simulink model "carTransStart"  (R2020a)
settings: Solver=ode23t  StartTime=0.0  StopTime=30  RelTol=1e-3  AbsTol=1e-3  EnableMultiTasking=on
libraries: nesl_utility x20, fl_lib x20, sdl_lib x17, simulink x1
settings Model: FPTRunName=Active  ExtModeAutoUpdateStatusClock=off  Creator=MathWorks  LastModifiedBy=SIDD N
settings SolverCC: AutoScaleAbsTol=off  ZcThreshold=0  ZeroCrossAlgorithm=Adaptive
settings DataIOCC: LimitDataPoints=on  SaveFormat=Array  SignalLoggingSaveFormat=ModelDataLogs  SaveOutput=off  SignalLogging=off  DSMLogging=off  SaveTime=off  ReturnWorkspaceOutputs=off
settings OptimizationCC: ExpressionDepthLimit=2147483647  InitFltsAndDblsToZero=on  LifeSpan=inf  BufferReusableBoundary=off
settings DebuggingCC: SaveWithParameterizedLinksMsg=none  UnderspecifiedInitializationDetection=Classic  MergeDetectMultiDrivingBlocksExec=none  SignalResolutionControl=TryResolveAllWithWarning  MultiTaskDSMMsg=warning  MultiTaskCondExecSysMsg=none  SigSpecEnsureSampleTimeMsg=none  FcnCallInpInsideContextMsg=warning  BusObjectLabelMismatch=none  StateNameClashWarn=warning  SFUnexpectedBacktrackingDiag=warning  SFNoUnconditionalDefaultTransitionDiag=warning  SFExecutionAtInitializationDiag=none  ArithmeticOperatorsInVariantConditions=warning
settings HardwareCC: ProdBitPerPointer=32  ProdBitPerSizeT=32  ProdBitPerPtrDiffT=32  ProdLargestAtomicFloat=None  ProdIntDivRoundTo=Undefined  ProdEndianess=Unspecified  ProdWordSize=32  ProdHWDeviceType=32-bit Generic  TargetBitPerPointer=64  TargetBitPerSizeT=64  TargetBitPerPtrDiffT=64  TargetLongLongMode=on  TargetIntDivRoundTo=Zero  TargetEndianess=LittleEndian  TargetWordSize=64  TargetHWDeviceType=MATLAB Host  ProdEqTarget=off
settings ModelReferenceCC: PropagateSignalLabelsOutOfModel=off
settings SFSimCC: SimUseLocalCustomCode=off  CustomCodeUndefinedFunction=UseInterfaceOnly
settings RTWCC: Description=Generic Real-Time Target  RTWUseLocalCustomCode=off
settings CodeAppCC: StateflowObjectComments=on
settings GRTTargetCC: TargetLangStandard=C89/C90 (ANSI)  CombineOutputUpdateFcns=off  GRTInterface=on
settings ConfigComp: CovMetricSettings=dw  CovHtmlReporting=on  CovSaveCumulativeToWorkspaceVar=on  CovSaveSingleToWorkspaceVar=on  CovExternalEMLEnable=off  CovSFcnEnable=off
settings SimscapeCC: SimscapeNormalizeSystem=off

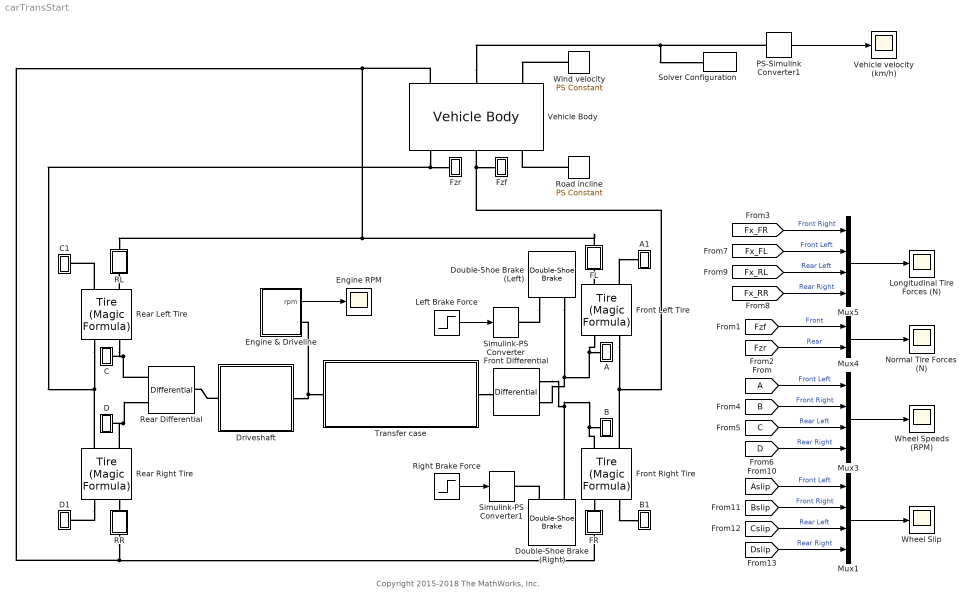
== system carTransStart ==
  note: Copyright 2015-2018 The MathWorks, Inc.
  A : Subsystem
  A1 : Subsystem
  B : Subsystem
  B1 : Subsystem
  C : Subsystem
  C1 : Subsystem
  D : Subsystem
  D1 : Subsystem
  Double-Shoe Brake (Left) : sdl_lib/Brakes & Detents/Rotational/Double-Shoe Brake  r_drum=200 mm  r_act=150 mm  r_pin=125 mm  theta_pin=15 deg  theta_0=5 deg  theta_shoe=120 deg  mu_visc=.01 N*m/(rad/s)  thermal_port=simscape.enum.thermaleffects.omit  mu=0.3  temperature_TLU=[280, 300, 320] K  mu_TLU=[.1, .05, .03]  thermal_mass=50 kJ/K  w_thr=0.01 rad/s  temperature_specify=off  temperature_priority=High  temperature=300 K  temperature_nominal_specify=off  temperature_nominal_unit=K  temperature_nominal_value=1
      settings: SourceProductBaseCode=LD  InternalSimscapePortConfiguration="{\"Bottom\":[],\"Left\":[{\"id\":\"F\",\"label\":\"F\",\"type\":\"input\"},{\"id\":\"S\",\"label\":\"S\",\"type\":\"foundation.mechanical.rotational.rotational\"}],\"Right\":[],\"Top\":[]}"
  Double-Shoe Brake (Right) : sdl_lib/Brakes & Detents/Rotational/Double-Shoe Brake  r_drum=200 mm  r_act=150 mm  r_pin=125 mm  theta_pin=15 deg  theta_0=5 deg  theta_shoe=120 deg  mu_visc=.01 N*m/(rad/s)  thermal_port=simscape.enum.thermaleffects.omit  mu=0.3  temperature_TLU=[280, 300, 320] K  mu_TLU=[.1, .05, .03]  thermal_mass=50 kJ/K  w_thr=0.01 rad/s  temperature_specify=off  temperature_priority=High  temperature=300 K  temperature_nominal_specify=off  temperature_nominal_unit=K  temperature_nominal_value=1
      settings: SourceProductBaseCode=LD  InternalSimscapePortConfiguration="{\"Bottom\":[],\"Left\":[{\"id\":\"F\",\"label\":\"F\",\"type\":\"input\"},{\"id\":\"S\",\"label\":\"S\",\"type\":\"foundation.mechanical.rotational.rotational\"}],\"Right\":[],\"Top\":[]}"
  Driveshaft : Subsystem
  Engine RPM : Scope
  Engine & Driveline : Subsystem
  FL : Subsystem
  FR : Subsystem
  Front Differential : sdl_lib/Gears/Differential  driveshaft_location=sdl.enum.differential_orientation.right  cd_ratio=4  friction_model=sdl.enum.gear_friction.none  mu_visc=[ 0 0 ] N*m/(rad/s)  efficiency=[ 0.85 0.92 ]  temperature_TLU=[ 280 300 320 ] K  efficiency_ss_TLU=[ 0.95 0.9 0.85 ]  efficiency_cd_TLU=[ 0.95 0.9 0.85 ]  pwr_thr=[.001, .001] W  thermal_mass=50 J/K  T_init=300 K  model_inertia=simscape.enum.onoff.off  carrier_inertia=0.001 kg*m^2  planet_inertia=0.001 kg*m^2
      settings: SourceProductBaseCode=LD
  Front Left Tire : sdl_lib/Tires & Vehicles/Tire (Magic Formula)  parameterization=1  F_z1=3000 N  F_x1=3500 N  kappa1=10  B_m=10  C_m=1.9  D_m=1  E_m=0.97  fz0=4e+3 N  p_Cx=1.685  p_Dx=[ 1.21 -0.037 ]  p_Ex=[ 0.344 0.095 -0.02 0 ]  p_Kx=[ 21.51 -0.163 0.245 ]  p_Hx=[ -0.002 0.002 ]  p_Vx=[ 0 0 ]  v_tr_thr=0.1 m/s  r_e=16*2.54/100 m  model_compliance=1  stiffness=200000 N/m  damping=1000 N/(m/s)  model_inertia=1  inertia=4.129 kg*m^2  initial_velocity=0 rpm  model_resistance=1  resistance_model=1  coeff=0.015  p_tire=250e3 Pa  alpha=-0.003  beta=0.97  coeff_a=84e-4  coeff_b=6.2e-4 s/m  coeff_c=1.6e-4 s^2/m^2  v_thr=1e-3 m/s
  Front Right Tire : sdl_lib/Tires & Vehicles/Tire (Magic Formula)  parameterization=1  F_z1=3000 N  F_x1=3500 N  kappa1=10  B_m=10  C_m=1.9  D_m=1  E_m=0.97  fz0=4e+3 N  p_Cx=1.685  p_Dx=[ 1.21 -0.037 ]  p_Ex=[ 0.344 0.095 -0.02 0 ]  p_Kx=[ 21.51 -0.163 0.245 ]  p_Hx=[ -0.002 0.002 ]  p_Vx=[ 0 0 ]  v_tr_thr=0.1 m/s  r_e=16*2.54/100 m  model_compliance=1  stiffness=200000 N/m  damping=1000 N/(m/s)  model_inertia=1  inertia=4.129 kg*m^2  initial_velocity=0 rpm  model_resistance=1  resistance_model=1  coeff=0.015  p_tire=250e3 Pa  alpha=-0.003  beta=0.97  coeff_a=84e-4  coeff_b=6.2e-4 s/m  coeff_c=1.6e-4 s^2/m^2  v_thr=1e-3 m/s
  Fzf : Subsystem
  Fzr : Subsystem
  Left Brake Force : Step  Time=10  After=1000  SampleTime=0
      settings: AttributesFormatString=Brake on @ %<Time> s
  Longitudinal Tire Forces (N) : Scope
  Mux1 : Mux
  Mux3 : Mux
  Mux4 : Mux  Inputs=2
  Mux5 : Mux
  Normal Tire Forces (N) : Scope
  PS-Simulink Converter1 : nesl_utility/PS-Simulink Converter  PhysicalDomain=network_engine_domain  SubClassName=ps_output  LeftPortType=input  RightPortType=output  PseudoPeriodic=off  Frequencies=[]  Unit=km/hr  AffineConversion=off
  RL : Subsystem
  RR : Subsystem
  Rear Differential : sdl_lib/Gears/Differential  driveshaft_location=2  cd_ratio=4  friction_model=1  mu_visc=[ 0 0 ] N*m/(rad/s)  efficiency=[ 0.85 0.92 ]  temperature_TLU=[ 280 300 320 ] K  efficiency_ss_TLU=[ 0.95 0.9 0.85 ]  efficiency_cd_TLU=[ 0.95 0.9 0.85 ]  pwr_thr=[.001, .001] W  thermal_mass=50 J/K  T_init=300 K  model_inertia=0  carrier_inertia=0.001 kg*m^2  planet_inertia=0.001 kg*m^2
      settings: SourceProductBaseCode=LD
  Rear Left Tire : sdl_lib/Tires & Vehicles/Tire (Magic Formula)  parameterization=1  F_z1=3000 N  F_x1=3500 N  kappa1=10  B_m=10  C_m=1.9  D_m=1  E_m=0.97  fz0=4e+3 N  p_Cx=1.685  p_Dx=[ 1.21 -0.037 ]  p_Ex=[ 0.344 0.095 -0.02 0 ]  p_Kx=[ 21.51 -0.163 0.245 ]  p_Hx=[ -0.002 0.002 ]  p_Vx=[ 0 0 ]  v_tr_thr=0.1 m/s  r_e=16*2.54/100 m  model_compliance=1  stiffness=200000 N/m  damping=1000 N/(m/s)  model_inertia=1  inertia=4.129 kg*m^2  initial_velocity=0 rpm  model_resistance=1  resistance_model=1  coeff=0.015  p_tire=250e3 Pa  alpha=-0.003  beta=0.97  coeff_a=84e-4  coeff_b=6.2e-4 s/m  coeff_c=1.6e-4 s^2/m^2  v_thr=1e-3 m/s
  Rear Right Tire : sdl_lib/Tires & Vehicles/Tire (Magic Formula)  parameterization=1  F_z1=3000 N  F_x1=3500 N  kappa1=10  B_m=10  C_m=1.9  D_m=1  E_m=0.97  fz0=4e+3 N  p_Cx=1.685  p_Dx=[ 1.21 -0.037 ]  p_Ex=[ 0.344 0.095 -0.02 0 ]  p_Kx=[ 21.51 -0.163 0.245 ]  p_Hx=[ -0.002 0.002 ]  p_Vx=[ 0 0 ]  v_tr_thr=0.1 m/s  r_e=16*2.54/100 m  model_compliance=1  stiffness=200000 N/m  damping=1000 N/(m/s)  model_inertia=1  inertia=4.129 kg*m^2  initial_velocity=0 rpm  model_resistance=1  resistance_model=1  coeff=0.015  p_tire=250e3 Pa  alpha=-0.003  beta=0.97  coeff_a=84e-4  coeff_b=6.2e-4 s/m  coeff_c=1.6e-4 s^2/m^2  v_thr=1e-3 m/s
  Right Brake Force : Step  Time=15  After=1000  SampleTime=0
      settings: AttributesFormatString=Brake on @ %<Time> s
  Road incline : fl_lib/Physical Signals/Sources/PS Constant  constant=pi*15/180
  Simulink-PS Converter : nesl_utility/Simulink-PS Converter  PhysicalDomain=network_engine_domain  SubClassName=ps_input  LeftPortType=input  RightPortType=output  PseudoPeriodic=off  Frequencies=[]  NoiseDistribution=none  NoiseParameters=[]  Unit=1  AffineConversion=off  FilteringAndDerivatives=zero  SimscapeFilterOrder=1  InputFilterTimeConstant=0.001  UdotUserProvided=1
  Simulink-PS Converter1 : nesl_utility/Simulink-PS Converter  PhysicalDomain=network_engine_domain  SubClassName=ps_input  LeftPortType=input  RightPortType=output  PseudoPeriodic=off  Frequencies=[]  NoiseDistribution=none  NoiseParameters=[]  Unit=1  AffineConversion=off  FilteringAndDerivatives=zero  SimscapeFilterOrder=1  InputFilterTimeConstant=0.001  UdotUserProvided=1
  Solver Configuration : nesl_utility/Solver Configuration  PhysicalDomain=network_engine_domain  SubClassName=solver  LeftPortType=input  RightPortType=generic  Tones=[]  Harmonics=[]  SimulateNoise=off  Profile=off  UseLocalSampling=off  EnableSwitchedLinearOptims=on  FrequencyDomain=off  UseCCode=off  RelTol=0.001  AbsTol=1e-06  MinStep=1e-09  ToWorkspace=off  RevertToSquareIcSolve=off  NumHomotopyIterations=100  PhasorMode=off  PhasorModeNumHarmonics=1  DoDC=off  ResidualTolerance=1e-9  UseLocalSolver=off  LocalSolverChoice=NE_BACKWARD_EULER_ADVANCER  LocalSolverSampleTime=0.1  DoFixedCost=off  MaxNonlinIter=3  MaxModeIter=2  LinearAlgebra=Sparse  EquationFormulation=NE_TIME_EF  DelaysMemoryBudget=1024  AutomaticFiltering=on  FilteringTimeConstant=0.001  PartitionStorageMethod=AS_NEEDED  PartitionMemoryBudget=1024  PartitionMethod=FAST
  Transfer case : Subsystem
  Vehicle Body : sdl_lib/Tires & Vehicles/Vehicle Body  mass=1500 kg  n_w=2  x_f=1.4 m  x_r=1.6 m  y_c=0.5 m  mass_var=simscape.enum.onoff.off  model_pitch=simscape.enum.onoff.off  inertia=4000 kg*m^2  suspension_model=sdl.enum.linearTLU.linear  k_f=1e4 N/m  b_f=1e4 N/(m/s)  k_r=1e4 N/m  b_r=1e4 N/(m/s)  k_f_TLU=[-2000, -1000, 0, 1000, 2000] N  x_f_TLU=[-.4, -.2, 0, .2, .4] m  b_f_TLU=[-200, -100, 0, 100, 200] N  v_f_TLU=[-4, -2, 0, 2, 4] m/s  k_r_TLU=[-2000, -1000, 0, 1000, 2000] N  x_r_TLU=[-.4, -.2, 0, .2, .4] m  b_r_TLU=[-200, -100, 0, 100, 200] N  v_r_TLU=[-4, -2, 0, 2, 4] m/s  interp_method=simscape.enum.interpolation.linear  extrap_method=simscape.enum.extrapolation.linear  model_hardstop=simscape.enum.onoff.off  upper_bound_f=.25 m  lower_bound_f=-.25 m  stop_k_f=1e6 N/m  stop_b_f=150 N/(m/s)  upper_bound_r=.25 m  lower_bound_r=-.25 m  stop_k_r=1e6 N/m  stop_b_r=150 N/(m/s)  initial_pitch=0 rad  initial_pitch_rate=0 rad/s  g=9.81 m/s^2  liftoff_warning=simscape.enum.onoff.off  area=3 m^2  Cd=0.4  rho=1.18 kg/m^3  v_specify=on  v_priority=High  v=0 m/s  v_nominal_specify=off  v_nominal_unit=m/s  v_nominal_value=1
  Vehicle velocity (km/h) : Scope
  Wheel Slip : Scope
  Wheel Speeds (RPM) : Scope
  Wind velocity : fl_lib/Physical Signals/Sources/PS Constant  constant=0
  wires:
  Engine & Driveline/1(rpm) -> Engine RPM/1
  PS-Simulink Converter1/1 -> Vehicle velocity (km/h)/1
  Left Brake Force/1 -> Simulink-PS Converter/1
  Right Brake Force/1 -> Simulink-PS Converter1/1
  Mux5/1 -> Longitudinal Tire Forces (N)/1
  Mux4/1 -> Normal Tire Forces (N)/1
  Mux3/1 -> Wheel Speeds (RPM)/1
  Mux1/1 -> Wheel Slip/1
  [A] -> Mux3/1  "Front Left"
  [B] -> Mux3/2  "Front Right"
  [C] -> Mux3/3  "Rear Left"
  [D] -> Mux3/4  "Rear Right"
  [Fzf] -> Mux4/1  "Front"
  [Fzr] -> Mux4/2  "Rear"
  [Fx_FR] -> Mux5/1  "Front Right"
  [Fx_FL] -> Mux5/2  "Front Left"
  [Fx_RR] -> Mux5/4  "Rear Right"
  [Fx_RL] -> Mux5/3  "Rear Left"
  [Aslip] -> Mux1/1  "Front Left"
  [Bslip] -> Mux1/2  "Front Right"
  [Cslip] -> Mux1/3  "Rear Left"
  [Dslip] -> Mux1/4  "Rear Right"
  connections:
  Rear Differential/RConn1 -- Rear Left Tire/LConn2 -- C/LConn1
  D/LConn1 -- Rear Right Tire/LConn2 -- Rear Differential/RConn2
  Double-Shoe Brake (Left)/LConn2 -- Front Differential/RConn1 -- A/LConn1 -- Front Left Tire/LConn2
  FL/RConn1 -- RL/RConn1 -- RR/RConn1 -- FR/RConn1 -- Vehicle Body/LConn1
  Front Right Tire/LConn1 -- Front Left Tire/LConn1 -- Vehicle Body/RConn2 -- Fzf/LConn1
  Vehicle Body/RConn1 -- Fzr/LConn1 -- Rear Right Tire/LConn1 -- Rear Left Tire/LConn1
  Road incline/RConn1 -- Vehicle Body/RConn3
  Wind velocity/RConn1 -- Vehicle Body/LConn3
  Vehicle Body/LConn2 -- PS-Simulink Converter1/LConn1 -- Solver Configuration/RConn1
  Front Right Tire/RConn2 -- FR/LConn1
  Rear Right Tire/RConn2 -- RR/LConn1
  Front Left Tire/RConn2 -- FL/LConn1
  Rear Left Tire/RConn2 -- RL/LConn1
  Front Left Tire/RConn1 -- A1/LConn1
  Front Right Tire/RConn1 -- B1/LConn1
  Rear Right Tire/RConn1 -- D1/LConn1
  Rear Left Tire/RConn1 -- C1/LConn1
  Double-Shoe Brake (Left)/LConn1 -- Simulink-PS Converter/RConn1
  Double-Shoe Brake (Right)/LConn1 -- Simulink-PS Converter1/RConn1
  Driveshaft/LConn1 -- Rear Differential/LConn1
  Driveshaft/RConn1 -- Engine & Driveline/RConn1 -- Transfer case/LConn1
  Front Right Tire/LConn2 -- Front Differential/RConn2 -- Double-Shoe Brake (Right)/LConn2 -- B/LConn1
  Transfer case/RConn1 -- Front Differential/LConn1

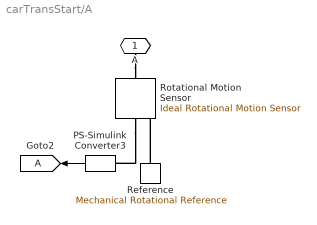
== system carTransStart/A ==
  PS-Simulink Converter3 : nesl_utility/PS-Simulink Converter  PhysicalDomain=network_engine_domain  SubClassName=ps_output  LeftPortType=input  RightPortType=output  PseudoPeriodic=off  Frequencies=[]  Unit=rpm  AffineConversion=off
  Reference : fl_lib/Mechanical/Rotational Elements/Mechanical Rotational Reference
  Rotational Motion Sensor : fl_lib/Mechanical/Mechanical Sensors/Ideal Rotational Motion Sensor  wrap_angle=simscape.enum.onoff.off  offset=0 rad
  A : PMIOPort  Side=Left
  tag scope: A=global
  wires:
  PS-Simulink Converter3/1 -> [A]
  connections:
  Rotational Motion Sensor/RConn2 -- PS-Simulink Converter3/LConn1
  Reference/LConn1 -- Rotational Motion Sensor/RConn1
  A/RConn1 -- Rotational Motion Sensor/LConn1

== system carTransStart/A1 ==
  PS-Simulink Converter : nesl_utility/PS-Simulink Converter  PhysicalDomain=network_engine_domain  SubClassName=ps_output  LeftPortType=input  RightPortType=output  PseudoPeriodic=off  Frequencies=[]  Unit=1  AffineConversion=off
  S : PMIOPort  Side=Left
  tag scope: Aslip=global
  wires:
  PS-Simulink Converter/1 -> [Aslip]
  connections:
  S/RConn1 -- PS-Simulink Converter/LConn1

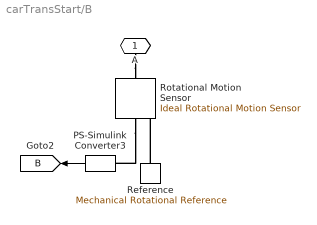
== system carTransStart/B ==
  PS-Simulink Converter3 : nesl_utility/PS-Simulink Converter  PhysicalDomain=network_engine_domain  SubClassName=ps_output  LeftPortType=input  RightPortType=output  PseudoPeriodic=off  Frequencies=[]  Unit=rpm  AffineConversion=off
  Reference : fl_lib/Mechanical/Rotational Elements/Mechanical Rotational Reference
  Rotational Motion Sensor : fl_lib/Mechanical/Mechanical Sensors/Ideal Rotational Motion Sensor  wrap_angle=simscape.enum.onoff.off  offset=0 rad
  A : PMIOPort  Side=Left
  tag scope: B=global
  wires:
  PS-Simulink Converter3/1 -> [B]
  connections:
  A/RConn1 -- Rotational Motion Sensor/LConn1
  Reference/LConn1 -- Rotational Motion Sensor/RConn1
  Rotational Motion Sensor/RConn2 -- PS-Simulink Converter3/LConn1

== system carTransStart/B1 ==
  PS-Simulink Converter : nesl_utility/PS-Simulink Converter  PhysicalDomain=network_engine_domain  SubClassName=ps_output  LeftPortType=input  RightPortType=output  PseudoPeriodic=off  Frequencies=[]  Unit=1  AffineConversion=off
  S : PMIOPort  Side=Left
  tag scope: Bslip=global
  wires:
  PS-Simulink Converter/1 -> [Bslip]
  connections:
  S/RConn1 -- PS-Simulink Converter/LConn1

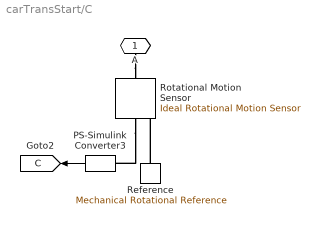
== system carTransStart/C ==
  PS-Simulink Converter3 : nesl_utility/PS-Simulink Converter  PhysicalDomain=network_engine_domain  SubClassName=ps_output  LeftPortType=input  RightPortType=output  PseudoPeriodic=off  Frequencies=[]  Unit=rpm  AffineConversion=off
  Reference : fl_lib/Mechanical/Rotational Elements/Mechanical Rotational Reference
  Rotational Motion Sensor : fl_lib/Mechanical/Mechanical Sensors/Ideal Rotational Motion Sensor  wrap_angle=simscape.enum.onoff.off  offset=0 rad
  A : PMIOPort  Side=Left
  tag scope: C=global
  wires:
  PS-Simulink Converter3/1 -> [C]
  connections:
  Rotational Motion Sensor/RConn2 -- PS-Simulink Converter3/LConn1
  Reference/LConn1 -- Rotational Motion Sensor/RConn1
  A/RConn1 -- Rotational Motion Sensor/LConn1

== system carTransStart/C1 ==
  PS-Simulink Converter : nesl_utility/PS-Simulink Converter  PhysicalDomain=network_engine_domain  SubClassName=ps_output  LeftPortType=input  RightPortType=output  PseudoPeriodic=off  Frequencies=[]  Unit=1  AffineConversion=off
  S : PMIOPort  Side=Left
  tag scope: Cslip=global
  wires:
  PS-Simulink Converter/1 -> [Cslip]
  connections:
  S/RConn1 -- PS-Simulink Converter/LConn1

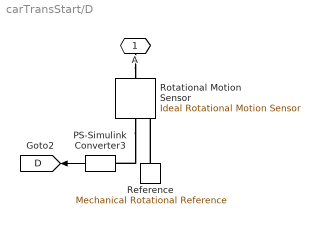
== system carTransStart/D ==
  PS-Simulink Converter3 : nesl_utility/PS-Simulink Converter  PhysicalDomain=network_engine_domain  SubClassName=ps_output  LeftPortType=input  RightPortType=output  PseudoPeriodic=off  Frequencies=[]  Unit=rpm  AffineConversion=off
  Reference : fl_lib/Mechanical/Rotational Elements/Mechanical Rotational Reference
  Rotational Motion Sensor : fl_lib/Mechanical/Mechanical Sensors/Ideal Rotational Motion Sensor  wrap_angle=simscape.enum.onoff.off  offset=0 rad
  A : PMIOPort  Side=Left
  tag scope: D=global
  wires:
  PS-Simulink Converter3/1 -> [D]
  connections:
  A/RConn1 -- Rotational Motion Sensor/LConn1
  Reference/LConn1 -- Rotational Motion Sensor/RConn1
  Rotational Motion Sensor/RConn2 -- PS-Simulink Converter3/LConn1

== system carTransStart/D1 ==
  PS-Simulink Converter : nesl_utility/PS-Simulink Converter  PhysicalDomain=network_engine_domain  SubClassName=ps_output  LeftPortType=input  RightPortType=output  PseudoPeriodic=off  Frequencies=[]  Unit=1  AffineConversion=off
  S : PMIOPort  Side=Left
  tag scope: Dslip=global
  wires:
  PS-Simulink Converter/1 -> [Dslip]
  connections:
  S/RConn1 -- PS-Simulink Converter/LConn1

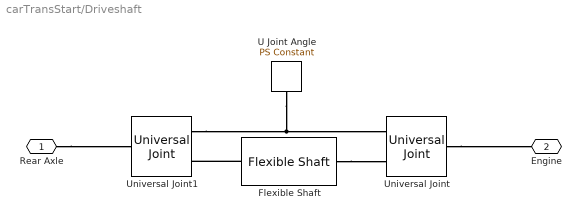
== system carTransStart/Driveshaft ==
  Flexible Shaft : sdl_lib/Couplings & Drives/Flexible Shaft  modelTransverse=simscape.enum.onoff.off  n_segments=1  parameterization=1  length=1 m  lengths=[1, .5, .25] m  shaft_stiffness=1e6 N*m/rad  shaft_inertia=0.02 kg*m^2  shaft_stiffnesses=[400000, 200000, 100000] N*m/rad  shaft_inertias=[.025, .02, .015] kg*m^2  eiIN=5e5 m^4*Pa  rhoaIN=19 kg/m  eiINs=[600000, 500000, 400000] m^4*Pa  rhoaINs=[20, 19, 18] kg/m  density=7.8e+3 kg/m^3  shear_modulus=7.93e+10 Pa  elastic_modulus=200e9 Pa  shaft_construction=1  diameter_outer=0.075 m  diameter_inner=0.05 m  diameter_outers=[.085, .075, .065] m  diameter_inners=[.055, .05, .045] m  damping_ratio=0.2  mu_visc_BF=[0, 0] N*m/(rad/s)  mu_visc=[ 0 0 ] N*m/(rad/s)  initial_deflection=0 rad  initial_velocity=0 rpm  num_supports=sdl.enum.num_supports.two  z_support=[0, 1] m  boundaryB1=sdl.enum.shaftSupport.clamp  DrotB1_row=[1000, 1000] N*m/(rad/s)  DtransB1_row=[20000, -44000, -44000, 350000] N/(m/s)  DtransB1_w_mat=[20000, -44000, -44000, 350000; 10000, -25000, -25000, 140000; 5000, -10000, -10000, 20000] N/(m/s)  KrotB1_row=[10000, 10000] N*m/rad  KtransB1_row=[1000000, -200000, -300000, 5000000] N/m  KtransB1_w_mat=[1000000, -600000, -3500000, 8000000; 1000000, -200000, -3000000, 5000000; 1000000, -50000, -2500000, 3000000] N/m  boundaryI1=sdl.enum.shaftSupport.clamp  DrotI1_row=[1000, 1000] N*m/(rad/s)  DtransI1_row=[20000, -44000, -44000, 350000] N/(m/s)  DtransI1_w_mat=[20000, -44000, -44000, 350000; 10000, -25000, -25000, 140000; 5000, -10000, -10000, 20000] N/(m/s)  KrotI1_row=[10000, 10000] N*m/rad  KtransI1_row=[1000000, -200000, -300000, 5000000] N/m  KtransI1_w_mat=[1000000, -600000, -3500000, 8000000; 1000000, -200000, -3000000, 5000000; 1000000, -50000, -2500000, 3000000] N/m  boundaryI2=sdl.enum.shaftSupport.clamp  DrotI2_row=[1000, 1000] N*m/(rad/s)  DtransI2_row=[20000, -44000, -44000, 350000] N/(m/s)  DtransI2_w_mat=[20000, -44000, -44000, 350000; 10000, -25000, -25000, 140000; 5000, -10000, -10000, 20000] N/(m/s)  KrotI2_row=[10000, 10000] N*m/rad  KtransI2_row=[1000000, -200000, -300000, 5000000] N/m  KtransI2_w_mat=[1000000, -600000, -3500000, 8000000; 1000000, -200000, -3000000, 5000000; 1000000, -50000, -2500000, 3000000] N/m  boundaryF1=sdl.enum.shaftSupport.clamp  DrotF1_row=[1000, 1000] N*m/(rad/s)  DtransF1_row=[20000, -44000, -44000, 350000] N/(m/s)  DtransF1_w_mat=[20000, -44000, -44000, 350000; 10000, -25000, -25000, 140000; 5000, -10000, -10000, 20000] N/(m/s)  KrotF1_row=[10000, 10000] N*m/rad  KtransF1_row=[1000000, -200000, -300000, 5000000] N/m  KtransF1_w_mat=[1000000, -600000, -3500000, 8000000; 1000000, -200000, -3000000, 5000000; 1000000, -50000, -2500000, 3000000] N/m  bearing_speed=[200, 500, 1500] rpm  alpha=10 1/s  beta=1e-8 s  noDisk=sdl.enum.shaftDisks.none  zDisk=0.5 m  mDiskIN=2 kg  IdDiskIN=0.025 kg*m^2  IpDiskIN=0.050 kg*m^2  offsetMR=[.01, .01] m*kg  offsetMassLocation=[.33, .67] m  offsetMR_initialAngleIN=[0, pi] rad  AnalysisMethod=sdl.enum.bendingAnalysisMethod.LumpedMass  ModeInputMethod=sdl.enum.modeInputMethod.SimscapeDetermined  numModesIn=6  mode_speed_dependency=sdl.enum.mode_speed_dependency.Static  OmegaNom=5000 rpm  wMax=1e8 rpm  dz=0.01 m  userMode_w=[280, 644, 615, 1285] rad/s  userMode_w_mat=[257, 780, 580, 1560; 280, 644, 615, 1285; 294, 513, 636, 1020] rad/s  userMode_z=[0, .1, .2, .3, .4, .5, .6, .7, .8, .9, 1] m  userMode_shapeX=[.1648, .0086, -.2759, .0162; .1671, .0093, -.2231, .0133; .1691, .01, -.1689, .0102; .1707, .0105, -.1135, .007; .1717, .0108, -.057, .0035; .1721, .0109, 0, 0; .1717, .0108, .057, -.0035; .1707, .0105, .1135, -.007; .1691, .01, .1689, -.0102; .1671, .0093, .2231, -.0133; .1648, .0086, .2759, -.0162]  userMode_shapeX_mat=cat(3, [.1842, .0134, -.3072, .0272; .1863, .0152, -.2482, .0226; .1882, .0169, -.1878, .0176; .1897, .0182, -.1261, .0121; .1906, .019, -.0634, .0062; .191, .0193, 0, 0; .1906, .019, .0634, -.0062; .1897, .0182, .1261, -.0121; .1882, .0169, .1878, -.0176; .1863, .0152, .2482, -.0226; .1842, .0134, .3072, -.0272], [.1648, .0086, -.2759, .0162; .1671, .0093, -.2231, .0133; .1691, .01, -.1689, .0102; .1707, .0105, -.1135, .007; .1717, .0108, -.057, .0035; .1721, .0109, 0, 0; .1717, .0108, .057, -.0035; .1707, .0105, .1135, -.007; .1691, .01, .1689, -.0102; .1671, .0093, .2231, -.0133; .1648, .0086, .2759, -.0162], [.1291, .0046, -.2166, .0082; .131, .0048, -.1751, .0067; .1327, .005, -.1327, .0051; .1341, .0052, -.0891, .0035; .135, .0053, -.0448, .0017; .1353, .0053, 0, 0; .135, .0053, .0448, -.0017; .1341, .0052, .0891, -.0035; .1327, .005, .1327, -.0051; .131, .0048, .1751, -.0067; .1291, .0046, .2166, -.0082])  userMode_shapeY=[.1193, -.1784, -.1997, -.3348; .1209, -.1933, -.1615, -.2751; .1224, -.2068, -.1223, -.2119; .1235, -.2176, -.0821, -.1445; .1243, -.2245, -.0413, -.0734; .1246, -.2269, 0, 0; .1243, -.2245, .0413, .0734; .1235, -.2176, .0821, .1445; .1224, -.2068, .1223, .2119; .1209, -.1933, .1615, .2751; .1193, -.1784, .1997, .3348]  userMode_shapeY_mat=cat(3, [.0885, -.1625, -.1475, -.3301; .0895, -.1847, -.1192, -.2745; .0904, -.2048, -.0902, -.2141; .0911, -.2209, -.0606, -.1475; .0916, -.2313, -.0304, -.0754; .0917, -.2349, 0, 0; .0916, -.2313, .0304, .0754; .0911, -.2209, .0606, .1475; .0904, -.2048, .0902, .2141; .0895, -.1847, .1192, .2745; .0885, -.1625, .1475, .3301], [.1193, -.1784, -.1997, -.3348; .1209, -.1933, -.1615, -.2751; .1224, -.2068, -.1223, -.2119; .1235, -.2176, -.0821, -.1445; .1243, -.2245, -.0413, -.0734; .1246, -.2269, 0, 0; .1243, -.2245, .0413, .0734; .1235, -.2176, .0821, .1445; .1224, -.2068, .1223, .2119; .1209, -.1933, .1615, .2751; .1193, -.1784, .1997, .3348], [.1566, -.1901, -.2628, -.3377; .1589, -.1994, -.2125, -.2753; .161, -.2079, -.1609, -.2103; .1627, -.2146, -.1081, -.1424; .1638, -.219, -.0544, -.0719; .1642, -.2205, 0, 0; .1638, -.219, .0544, .0719; .1627, -.2146, .1081, .1424; .161, -.2079, .1609, .2103; .1589, -.1994, .2125, .2753; .1566, -.1901, .2628, .3377])
      settings: SourceProductBaseCode=LD  InternalSimscapePortConfiguration="{\"Bottom\":[],\"Left\":[{\"id\":\"B\",\"label\":\"B\",\"type\":\"foundation.mechanical.rotational.rotational\"}],\"Right\":[{\"id\":\"F\",\"label\":\"F\",\"type\":\"foundation.mechanical.rotational.rotational\"}],\"Top\":[]}"
  U Joint Angle : fl_lib/Physical Signals/Sources/PS Constant  constant=15*pi/180
  Universal Joint : sdl_lib/Couplings & Drives/Universal Joint  Amax=pi / 4 rad  compliance=1  k=1e6 N*m/rad  b=1e3 N*m/(rad/s)  thetaB0=0 rad  t0=0 N*m
      settings: SourceProductBaseCode=LD  InternalSimscapePortConfiguration="{\"Bottom\":[],\"Left\":[{\"id\":\"A\",\"label\":\"A\",\"type\":\"input\"},{\"id\":\"B\",\"label\":\"B\",\"type\":\"foundation.mechanical.rotational.rotational\"}],\"Right\":[{\"id\":\"F\",\"label\":\"F\",\"type\":\"foundation.mechanical.rotational.rotational\"}],\"Top\":[]}"
  Universal Joint1 : sdl_lib/Couplings & Drives/Universal Joint  Amax=pi / 4 rad  compliance=1  k=1e6 N*m/rad  b=1e3 N*m/(rad/s)  thetaB0=0 rad  t0=0 N*m
      settings: SourceProductBaseCode=LD  InternalSimscapePortConfiguration="{\"Bottom\":[],\"Left\":[{\"id\":\"A\",\"label\":\"A\",\"type\":\"input\"},{\"id\":\"B\",\"label\":\"B\",\"type\":\"foundation.mechanical.rotational.rotational\"}],\"Right\":[{\"id\":\"F\",\"label\":\"F\",\"type\":\"foundation.mechanical.rotational.rotational\"}],\"Top\":[]}"
  Rear Axle : PMIOPort  Side=Left
  Engine : PMIOPort  Port=2  Side=Right
  connections:
  Universal Joint/RConn1 -- Engine/RConn1
  Rear Axle/RConn1 -- Universal Joint1/RConn1
  U Joint Angle/RConn1 -- Universal Joint/LConn1 -- Universal Joint1/LConn1
  Flexible Shaft/RConn1 -- Universal Joint/LConn2
  Flexible Shaft/LConn1 -- Universal Joint1/LConn2

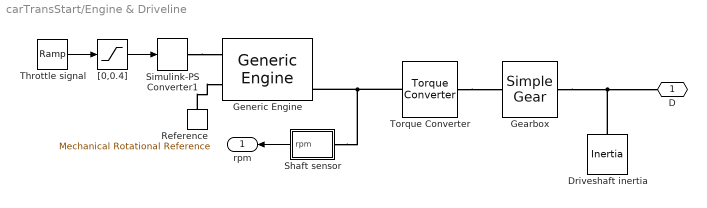
== system carTransStart/Engine & Driveline ==
  Driveshaft inertia : fl_lib/Mechanical/Rotational Elements/Inertia  inertia=12 kg*m^2  w_specify=off  w_priority=High  w=0 rad/s  w_nominal_specify=off  w_nominal_unit=rad/s  w_nominal_value=1  t_specify=off  t_priority=High  t=0 N*m  t_nominal_specify=off  t_nominal_unit=N*m  t_nominal_value=1
  Gearbox : sdl_lib/Gears/Simple Gear  ratio=2  rotation_direction=1  friction_model=1  T_noload=0.1 N*m  T_nom=5 N*m  efficiency_nom=0.8  efficiency=0.8  mu_visc=[ 0 0 ] N*m/(rad/s)  w_thr=0.01 rad/s  pwr_thr=0.001 W  enable_faults=simscape.enum.onoff.off  efficiency_fault=0.05  external_fault=simscape.enum.onoff.off  temporal_fault=simscape.enum.onoff.off  fault_time=5 s  fault_angles=pi / 12 rad  report_fault=1  temperature_TLU=[ 280 300 320 ] K  load_TLU=[ 1 5 10 ] N*m  efficiency_TLU=[ 0.95 0.9 0.85 ]  efficiency_TLU2=[ 0.85 0.8 0.75; 0.95 0.9 0.85; 0.85 0.8 0.7 ]  thermal_mass=50 J/K  T_init=300 K
  Generic Engine : sdl_lib/Engines/Generic Engine  model_parameterization=1  engine_type=1  P_max=150e3 W  w_P_max=4500 rpm  w_max=6000 rpm  w_min=500 rpm  w_tab=[ 500 1000 2e+3 3e+3 4e+3 5e+3 6e+3 7e+3 ] rpm  trq_tab=[ 380 380 380 380 350 280 200 80 ] N*m  pwr_tab=[ 2e+4 4e+4 7.8e+4 1.2e+5 1.45e+5 1.48e+5 1.25e+5 6e+4 ] W  interp_method=1  model_inertia=1  inertia=0.2 kg*m^2  initial_velocity=800 rpm  model_time_constant=0  time_constant=0.2 s  T0=0  w_thr=100 rpm  idle_speed=0  idle_speed_reference=1000 rpm  tau_controller=1 s  idle_w_thr=1 rpm  redline=0  redline_speed=5000 rpm  tau_redline=1 s  redline_w_thr=1 rpm  fc_model=1  fc_per_rev=25 mg/rev  displaced_volume=400 cm^3  rev_per_cycle=2  fc_w_tab=[ 1000 2e+3 3e+3 4e+3 5e+3 6e+3 ] rpm  fc_trq_tab=[ 0 80 160 200 240 320 360 400 ] N*m  fc_tab=[ 0.5 0.9 1.4 1.6 1.9 2.7 3.4 4.4; 1 1.7 2.7 3.1 3.6 5 6 7.4; 1.4 2.7 4 4.8 5.6 7.5 8.5 10.5; 2 3.6 5.8 6.7 8 10.4 11.7 13.3; 2.5 4.8 7.9 9.4 10.8 14 16.2 18.6; 3.1 6 10.3 11.9 13.8 18.4 22 26.5 ] g/s  bmep_tab=[ 0 250 500 625 750 1000 1.15e+3 1.25e+3 ] kPa  bsfc_tab=[ 410 380 300 280 270 290 320 380; 410 370 290 270 260 270 285 320; 415 380 290 275 265 270 270 300; 420 390 310 290 285 280 280 285; 430 410 340 320 310 300 310 320; 450 430 370 340 330 330 350 380 ] g/hr/kW  fc_interp_method=1
      settings: SourceProductBaseCode=LD  InternalSimscapePortConfiguration="{\"Bottom\":[],\"Left\":[{\"id\":\"T\",\"label\":\"T\",\"type\":\"input\"},{\"id\":\"B\",\"label\":\"B\",\"type\":\"foundation.mechanical.rotational.rotational\"}],\"Right\":[{\"id\":\"P\",\"label\":\"P\",\"type\":\"output\"},{\"id\":\"FC\",\"label\":\"FC\",\"type\":\"output\"},{\"id\":\"F\",\"label\":\"F\",\"type\":\"foundation.mechanical.rotational.rotational\"}],\"Top\":[]}"
  Reference : fl_lib/Mechanical/Rotational Elements/Mechanical Rotational Reference
  Shaft sensor : Subsystem
  Simulink-PS Converter1 : nesl_utility/Simulink-PS Converter  PhysicalDomain=network_engine_domain  SubClassName=ps_input  LeftPortType=input  RightPortType=output  PseudoPeriodic=off  Frequencies=[]  NoiseDistribution=none  NoiseParameters=[]  Unit=1  AffineConversion=off  FilteringAndDerivatives=zero  SimscapeFilterOrder=1  InputFilterTimeConstant=.001  UdotUserProvided=0
  Throttle signal : simulink/Sources/Ramp  slope=0.9/2  start=0  InitialOutput=0.02
  Torque Converter : sdl_lib/Couplings & Drives/Torque Converter  n_vector=[0 0.50 0.60 0.70 0.80 0.87 0.92 0.94 0.96 0.97]  trq_vector=[2.2320 1.5462 1.4058 1.2746 1.1528 1.0732 1.0192 0.9983 0.9983 0.9983]  cf_vector_parameterization=1  cf_vector_reference_speed=1  cf_vector=[12.2938 12.8588 13.1452 13.6285 14.6163 16.2675 19.3503 22.1046 29.9986 50.00] (rad/s)/(N*m)^0.5  cf_vector_sq=1e-3*[ 6.616 6.048 5.787 5.384 4.681 3.779 2.671 2.047 1.111 0.400] N*m/(rad/s)^2  interp_method=1  extrap_method=1  model_lag=0  tau=0.02 s  initial_trq_ratio=0
      settings: SourceProductBaseCode=LD  InternalSimscapePortConfiguration="{\"Bottom\":[],\"Left\":[{\"id\":\"I\",\"label\":\"I\",\"type\":\"foundation.mechanical.rotational.rotational\"}],\"Right\":[{\"id\":\"T\",\"label\":\"T\",\"type\":\"foundation.mechanical.rotational.rotational\"}],\"Top\":[]}"
  "[0,0.4]" : Saturate  UpperLimit=0.4  LowerLimit=0
  D : PMIOPort  Side=Right
  rpm : Outport  VectorParamsAs1DForOutWhenUnconnected=off
  wires:
  Shaft sensor/1(rpm) -> rpm/1
  Throttle signal/1 -> "[0,0.4]"/1
  "[0,0.4]"/1 -> Simulink-PS Converter1/1
  connections:
  Torque Converter/LConn1 -- Shaft sensor/LConn1 -- Generic Engine/RConn3
  Reference/LConn1 -- Generic Engine/LConn2
  Simulink-PS Converter1/RConn1 -- Generic Engine/LConn1
  Driveshaft inertia/LConn1 -- D/RConn1 -- Gearbox/RConn1
  Torque Converter/RConn1 -- Gearbox/LConn1

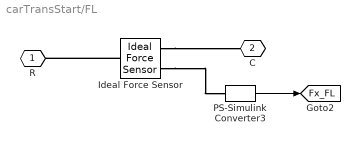
== system carTransStart/FL ==
  Ideal Force Sensor : fl_lib/Mechanical/Mechanical Sensors/Ideal Force Sensor
  PS-Simulink Converter3 : nesl_utility/PS-Simulink Converter  PhysicalDomain=network_engine_domain  SubClassName=ps_output  LeftPortType=input  RightPortType=output  PseudoPeriodic=off  Frequencies=[]  Unit=N  AffineConversion=off
  R : PMIOPort  Side=Left
  C : PMIOPort  Port=2  Side=Right
  tag scope: Fx_FL=global
  wires:
  PS-Simulink Converter3/1 -> [Fx_FL]
  connections:
  Ideal Force Sensor/LConn1 -- R/RConn1
  Ideal Force Sensor/RConn1 -- C/RConn1
  Ideal Force Sensor/RConn2 -- PS-Simulink Converter3/LConn1

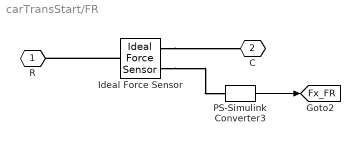
== system carTransStart/FR ==
  Ideal Force Sensor : fl_lib/Mechanical/Mechanical Sensors/Ideal Force Sensor
  PS-Simulink Converter3 : nesl_utility/PS-Simulink Converter  PhysicalDomain=network_engine_domain  SubClassName=ps_output  LeftPortType=input  RightPortType=output  PseudoPeriodic=off  Frequencies=[]  Unit=N  AffineConversion=off
  R : PMIOPort  Side=Left
  C : PMIOPort  Port=2  Side=Right
  tag scope: Fx_FR=global
  wires:
  PS-Simulink Converter3/1 -> [Fx_FR]
  connections:
  Ideal Force Sensor/RConn2 -- PS-Simulink Converter3/LConn1
  Ideal Force Sensor/RConn1 -- C/RConn1
  Ideal Force Sensor/LConn1 -- R/RConn1

== system carTransStart/Fzf ==
  PS-Simulink Converter3 : nesl_utility/PS-Simulink Converter  PhysicalDomain=network_engine_domain  SubClassName=ps_output  LeftPortType=input  RightPortType=output  PseudoPeriodic=off  Frequencies=[]  Unit=N  AffineConversion=off
  f : PMIOPort  Side=Left
  tag scope: Fzf=global
  wires:
  PS-Simulink Converter3/1 -> [Fzf]
  connections:
  f/RConn1 -- PS-Simulink Converter3/LConn1

== system carTransStart/Fzr ==
  PS-Simulink Converter3 : nesl_utility/PS-Simulink Converter  PhysicalDomain=network_engine_domain  SubClassName=ps_output  LeftPortType=input  RightPortType=output  PseudoPeriodic=off  Frequencies=[]  Unit=N  AffineConversion=off
  f : PMIOPort  Side=Left
  tag scope: Fzr=global
  wires:
  PS-Simulink Converter3/1 -> [Fzr]
  connections:
  f/RConn1 -- PS-Simulink Converter3/LConn1

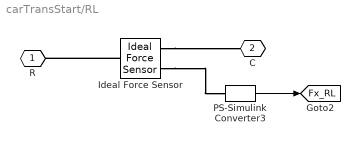
== system carTransStart/RL ==
  Ideal Force Sensor : fl_lib/Mechanical/Mechanical Sensors/Ideal Force Sensor
  PS-Simulink Converter3 : nesl_utility/PS-Simulink Converter  PhysicalDomain=network_engine_domain  SubClassName=ps_output  LeftPortType=input  RightPortType=output  PseudoPeriodic=off  Frequencies=[]  Unit=N  AffineConversion=off
  R : PMIOPort  Side=Left
  C : PMIOPort  Port=2  Side=Right
  tag scope: Fx_RL=global
  wires:
  PS-Simulink Converter3/1 -> [Fx_RL]
  connections:
  Ideal Force Sensor/RConn2 -- PS-Simulink Converter3/LConn1
  Ideal Force Sensor/RConn1 -- C/RConn1
  Ideal Force Sensor/LConn1 -- R/RConn1

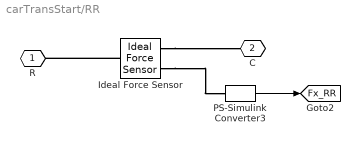
== system carTransStart/RR ==
  Ideal Force Sensor : fl_lib/Mechanical/Mechanical Sensors/Ideal Force Sensor
  PS-Simulink Converter3 : nesl_utility/PS-Simulink Converter  PhysicalDomain=network_engine_domain  SubClassName=ps_output  LeftPortType=input  RightPortType=output  PseudoPeriodic=off  Frequencies=[]  Unit=N  AffineConversion=off
  R : PMIOPort  Side=Left
  C : PMIOPort  Port=2  Side=Right
  tag scope: Fx_RR=global
  wires:
  PS-Simulink Converter3/1 -> [Fx_RR]
  connections:
  Ideal Force Sensor/LConn1 -- R/RConn1
  Ideal Force Sensor/RConn1 -- C/RConn1
  Ideal Force Sensor/RConn2 -- PS-Simulink Converter3/LConn1

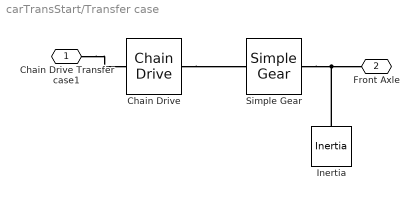
== system carTransStart/Transfer case ==
  "Chain Drive " : sdl_lib/Couplings & Drives/Chain Drive  chain_model=sdl.enum.chain_model.flexible  radius_a=80 mm  radius_b=40 mm  slack=50 mm  k_chain=100000 N/m  mu_visc_chain=5 N/(m/s)  mu_visc_a=0.001 N*m/(rad/s)  mu_visc_b=0.001 N*m/(rad/s)  breakable=sdl.enum.max_tension.off  F_max=1e6 N  x_specify=off  x_priority=High  x=0 mm  x_nominal_specify=off  x_nominal_unit=mm  x_nominal_value=1
      settings: SourceProductBaseCode=LD  InternalSimscapePortConfiguration="{\"Bottom\":[],\"Left\":[{\"id\":\"A\",\"label\":\"A\",\"type\":\"foundation.mechanical.rotational.rotational\"}],\"Right\":[{\"id\":\"B\",\"label\":\"B\",\"type\":\"foundation.mechanical.rotational.rotational\"}],\"Top\":[]}"
  Inertia : fl_lib/Mechanical/Rotational Elements/Inertia  inertia=0.01 kg*m^2  w_specify=off  w_priority=High  w=0 rad/s  w_nominal_specify=off  w_nominal_unit=rad/s  w_nominal_value=1  t_specify=off  t_priority=None  t=0 N*m  t_nominal_specify=off  t_nominal_unit=N*m  t_nominal_value=1
  Simple Gear : sdl_lib/Gears/Simple Gear  ratio=2  rotation_direction=1  friction_model=sdl.enum.gear_efficiencies_load.off  T_noload=0.1 N*m  T_nom=5 N*m  efficiency_nom=0.8  efficiency=0.8  mu_visc=[0, 0] N*m/(rad/s)  w_thr=0.01 rad/s  pwr_thr=0.001 W  enable_faults=simscape.enum.onoff.off  efficiency_fault=0.05  external_fault=simscape.enum.onoff.off  temporal_fault=simscape.enum.onoff.off  fault_time=5 s  fault_angles=pi / 12 rad  report_fault=1  temperature_TLU=[280, 300, 320] K  load_TLU=[1, 5, 10] N*m  efficiency_TLU=[.95, .9, .85]  efficiency_TLU2=[.85, .8, .75; .95, .9, .85; .85, .8, .7]  thermal_mass=50 J/K  T_init=300 K
  Chain Drive Transfer case1 : PMIOPort  Side=Left
  Front Axle : PMIOPort  Port=2  Side=Right
  connections:
  "Chain Drive "/RConn1 -- Simple Gear/LConn1
  Chain Drive Transfer case1/RConn1 -- "Chain Drive "/LConn1
  Simple Gear/RConn1 -- Front Axle/RConn1 -- Inertia/LConn1

== system carTransStart/Engine & Driveline/Shaft sensor ==
  PS-Simulink Converter3 : nesl_utility/PS-Simulink Converter  PhysicalDomain=network_engine_domain  SubClassName=ps_output  LeftPortType=input  RightPortType=output  PseudoPeriodic=off  Frequencies=[]  Unit=rpm  AffineConversion=off
  Reference : fl_lib/Mechanical/Rotational Elements/Mechanical Rotational Reference
  Rotational Motion Sensor : fl_lib/Mechanical/Mechanical Sensors/Ideal Rotational Motion Sensor  wrap_angle=simscape.enum.onoff.off  offset=0 rad
  R : PMIOPort  Side=Left
  rpm : Outport  VectorParamsAs1DForOutWhenUnconnected=off
  wires:
  PS-Simulink Converter3/1 -> rpm/1
  connections:
  R/RConn1 -- Rotational Motion Sensor/LConn1
  Reference/LConn1 -- Rotational Motion Sensor/RConn1
  Rotational Motion Sensor/RConn2 -- PS-Simulink Converter3/LConn1
